simulink model "gnu_radio_rx"  (R2014b)
settings: Solver=ode45  StartTime=0.0  StopTime=inf  RelTol=1e-3
libraries: siglabs_lib x1, dspnetwork x1
settings Model: Creator=Ben  LastModifiedBy=Ben

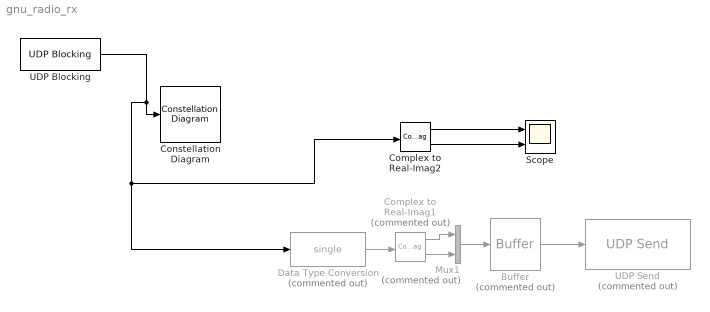
== system gnu_radio_rx ==
  Buffer : Buffer  Commented=on  N=180  TreatMby1Signals=One channel
  Complex to Real-Imag1 : ComplexToRealImag  Commented=on
  Complex to Real-Imag2 : ComplexToRealImag
  Constellation Diagram : ConstellationDiagram
  Data Type Conversion : DataTypeConversion  Commented=on  OutDataTypeStr=single
  Mux1 : Mux  Commented=on  Inputs=2
  Scope : Scope  NumInputPorts=2
      settings: YMin=-1~-1  YMax=1~1
  UDP Blocking : siglabs_lib/UDP Blocking  sample_time=1/1000
  UDP Send : dspnetwork/UDP Send  Commented=on  remoteURL='192.168.1.24'  remotePort=1234  localURL='0.0.0.0'  localPortSource=Automatically determine  localPort=-1  sampletime=-1  separateLengthPort=0
  wires:
  UDP Blocking/1 -> Complex to Real-Imag2/1, Data Type Conversion/1, Constellation Diagram/1
  Data Type Conversion/1 -> Complex to Real-Imag1/1
  Complex to Real-Imag1/1 -> Mux1/1
  Complex to Real-Imag1/2 -> Mux1/2
  Mux1/1 -> Buffer/1
  Buffer/1 -> UDP Send/1
  Complex to Real-Imag2/1 -> Scope/1
  Complex to Real-Imag2/2 -> Scope/2
